simulink model "delay_brake"  (R2021a)
settings: Solver=FixedStepAuto  StartTime=0.0  StopTime=inf  FixedStep=0.05  RelTol=1e-3
undefined symbols (not defined in the file): Linear
libraries: robotlib x16
settings Model: Creator=ivory  LastModifiedBy=vanderbilt
settings SolverCC: AlgebraicLoopSolver=TrustRegion
settings OptimizationCC: EnhancedBackFolding=on  PassReuseOutputArgsAs=Individual arguments  ZeroExternalMemoryAtStartup=off  ZeroInternalMemoryAtStartup=off  MaxStackSize=64  OptimizeBlockOrder=speed  DifferentSizesBufferReuse=on  OptimizationCustomize=off  EfficientTunableParamExpr=on
settings DebuggingCC: ParameterTunabilityLossMsg=error  SFMachineParentedDataDiag=warning
settings HardwareCC: ProdBitPerPointer=32  ProdBitPerSizeT=32  ProdBitPerPtrDiffT=32  ProdLargestAtomicFloat=None  ProdIntDivRoundTo=Undefined  ProdEndianess=Unspecified  ProdWordSize=32  ProdHWDeviceType=Generic->Unspecified (assume 32-bit Generic)
settings SFSimCC: MATLABDynamicMemAlloc=off  SimTargetLang=C++
settings RTWCC: SystemTargetFile=ert.tlc  HardwareBoard=Robot Operating System (ROS)  TLCOptions="-aInlineSetEventsForThisBaseRateFcn=TLC_FALSE -aSuppressMultiTaskScheduler=TLC_FALSE  -aRateBasedStepFcn=0"  TemplateMakefile=ert_default_tmf  GenerateReport=on  Toolchain=Catkin  IncludeHyperlinkInReport=on  LaunchReport=on  TargetLang=C++  GenerateTraceInfo=on  GenerateTraceReport=on  GenerateTraceReportSl=on  GenerateTraceReportSf=on  GenerateTraceReportEml=on
settings CodeAppCC: ForceParamTrailComments=on  IgnoreCustomStorageClasses=off  OperatorAnnotations=on  SimulinkDataObjDesc=on  SFDataObjDesc=on  InsertBlockDesc=on
settings ERTTargetCC: SupportContinuousTime=on  SupportVariableSizeSignals=on

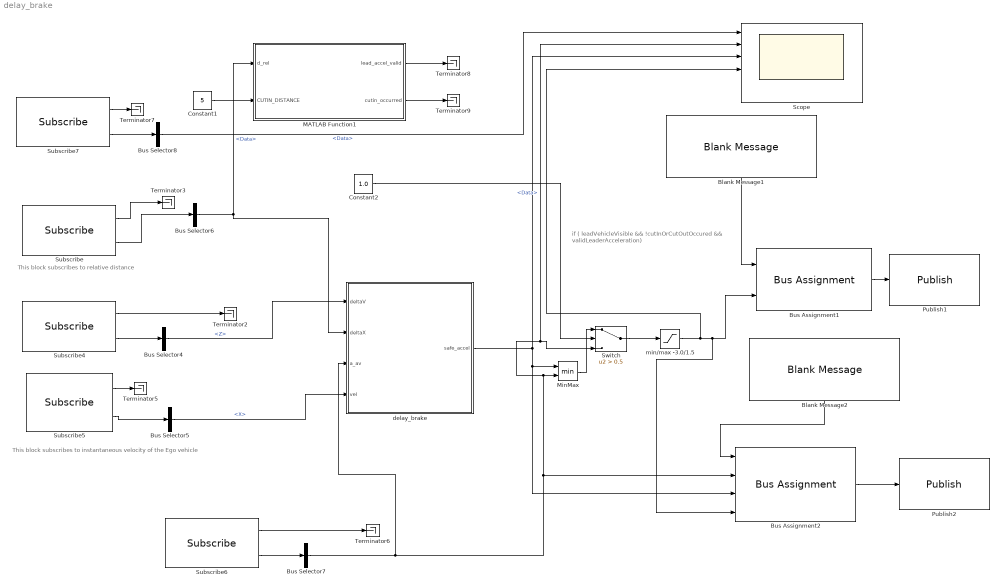
== system delay_brake ==
  note: if ( leadVehicleVisible && !cutInOrCutOutOccured && validLeaderAcceleration)
  note: This block subscribes
      | to relative distance
  note: This block subscribes to
      | instantaneous velocity of the Ego vehicle
  Blank Message1 : robotlib/Blank Message  messageClass=Message  entityType=std_msgs/Float64  messageType=std_msgs/Float64  SampleTime=inf  legacyBusStruct=off
  Blank Message2 : robotlib/Blank Message  messageClass=Message  entityType=geometry_msgs/Twist  messageType=geometry_msgs/Twist  SampleTime=inf  legacyBusStruct=off
  Bus Assignment1 : BusAssignment  AssignedSignals=Data
  Bus Assignment2 : BusAssignment  AssignedSignals=Linear.X,Linear.Y,Linear.Z
  Bus Selector4 : BusSelector  OutputSignals=Linear.Z
  Bus Selector5 : BusSelector  OutputSignals=Linear.X
  Bus Selector6 : BusSelector  OutputSignals=Data
  Bus Selector7 : BusSelector  OutputSignals=Data
  Bus Selector8 : BusSelector  OutputSignals=Data
  Constant1 : Constant  Value=5
  Constant2 : Constant  Value=1.0
  MATLAB Function1 : MATLAB Function  TreatAsAtomicUnit=on
  MinMax : MinMax  Inputs=2
  Publish1 : robotlib/Publish  topicSource=Specify your own  topic=cmd_accel  messageType=std_msgs/Float64  legacyBusStruct=off  messageQueueLength=1
  Publish2 : robotlib/Publish  topicSource=Specify your own  topic=/delay_brake/delay_brake_debug  messageType=geometry_msgs/Twist  legacyBusStruct=off  messageQueueLength=1
  Scope : Scope  NumInputPorts=6
  Subscribe : robotlib/Subscribe  topicSource=Specify your own  topic=lead_dist  messageType=std_msgs/Float64  SampleTime=-1  legacyBusStruct=off  messageQueueLength=1
  Subscribe4 : robotlib/Subscribe  topicSource=Specify your own  topic=rel_vel  messageType=geometry_msgs/Twist  SampleTime=-1  legacyBusStruct=off  messageQueueLength=1
  Subscribe5 : robotlib/Subscribe  topicSource=Specify your own  topic=vel  messageType=geometry_msgs/Twist  SampleTime=-1  legacyBusStruct=off  messageQueueLength=1
  Subscribe6 : robotlib/Subscribe  topicSource=Specify your own  topic=cmd_accel_pre  messageType=std_msgs/Float64  SampleTime=-1  legacyBusStruct=off  messageQueueLength=1
  Subscribe7 : robotlib/Subscribe  topicSource=Specify your own  topic=/car/hud/mini_car_enable  messageType=std_msgs/Bool  SampleTime=-1  legacyBusStruct=off  messageQueueLength=1
  Switch : Switch  Criteria=u2 > Threshold  Threshold=0.5
  Terminator{2..3,5..9} (7 alike) : Terminator
  delay_brake : Subsystem
  min/max -3.0/1.5 : Saturate  UpperLimit=1.5  LowerLimit=-3.0
  wires:
  Subscribe4/1 -> Terminator2/1
  Bus Selector4/1 -> delay_brake/1(deltaV)  "<Z>"
  Subscribe5/2 -> Bus Selector5/1
  Subscribe4/2 -> Bus Selector4/1
  Bus Selector5/1 -> delay_brake/4(vel)  "<X>"
  Bus Assignment1/1 -> Publish1/1
  Blank Message1/1 -> Bus Assignment1/1
  Subscribe5/1 -> Terminator5/1
  Subscribe/1 -> Terminator3/1
  Subscribe/2 -> Bus Selector6/1
  Bus Selector6/1 -> MATLAB Function1/1(d_rel), delay_brake/2(deltaX)  "<Data>"
  Subscribe6/2 -> Bus Selector7/1
  Bus Selector7/1 -> delay_brake/3(a_av), MinMax/2, Switch/3, Scope/2, Bus Assignment2/2  "<Data>"
  Subscribe6/1 -> Terminator6/1
  Subscribe7/2 -> Bus Selector8/1
  Subscribe7/1 -> Terminator7/1
  Bus Selector8/1 -> Scope/1  "<Data>"
  Constant1/1 -> MATLAB Function1/2(CUTIN_DISTANCE)
  delay_brake/1(safe_accel) -> Scope/3, Bus Assignment2/3, MinMax/1
  MinMax/1 -> Switch/1
  min/max -3.0/1.5/1 -> Scope/4, Bus Assignment2/4, Bus Assignment1/2
  Blank Message2/1 -> Bus Assignment2/1
  Bus Assignment2/1 -> Publish2/1
  MATLAB Function1/1(lead_accel_valid) -> Terminator8/1
  MATLAB Function1/2(cutin_occurred) -> Terminator9/1
  Switch/1 -> min/max -3.0/1.5/1
  Constant2/1 -> Switch/2

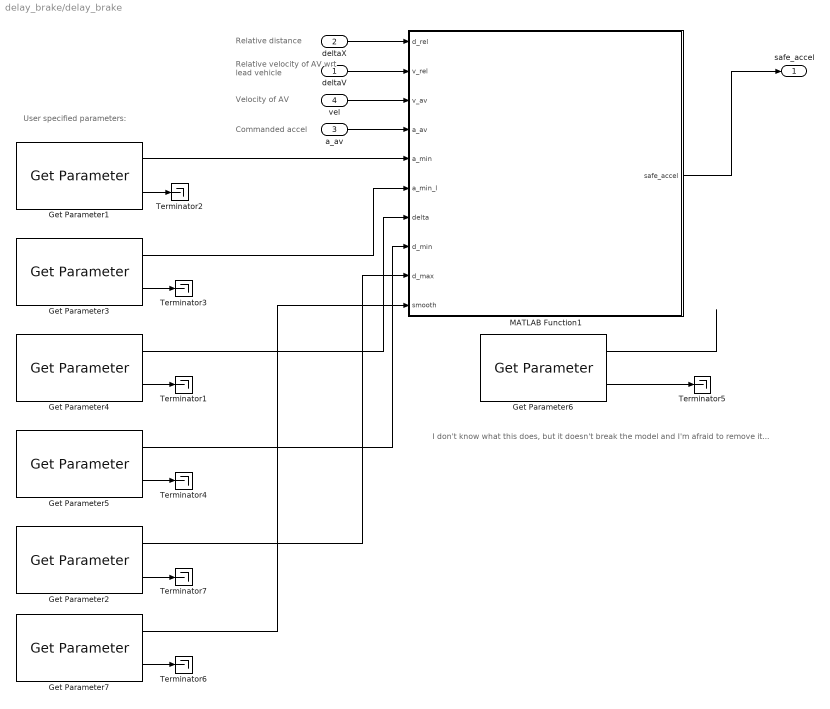
== system delay_brake/delay_brake ==
  note: I don't know what this does, but it doesn't break the model and I'm afraid to remove it...
  note: Velocity of AV
  note: Relative velocity of
      | AV wrt lead vehicle
  note: Relative distance
  note: Commanded accel
  note: User specified parameters:
  deltaV : Inport
  deltaX : Inport  Port=2
  a_av : Inport  Port=3
  vel : Inport  Port=4
  Get Parameter1 : robotlib/Get Parameter  ParameterSource=Specify your own  ParameterName=a_min  ParameterType=double  ParameterMaxArrayLength=16  ParameterInitialValue=-3.0  SampleTime=-1  ShowErrorCodeOutput=on  ModelName=delay_brake  BlockId=ParamGet_delay_brake_447
      settings: SourceProductBaseCode=RR
  Get Parameter2 : robotlib/Get Parameter  ParameterSource=Specify your own  ParameterName=d_max  ParameterType=double  ParameterMaxArrayLength=16  ParameterInitialValue=15.0  SampleTime=-1  ShowErrorCodeOutput=on  ModelName=delay_brake  BlockId=ParamGet_delay_brake_448
      settings: SourceProductBaseCode=RR
  Get Parameter3 : robotlib/Get Parameter  ParameterSource=Specify your own  ParameterName=a_min_l  ParameterType=double  ParameterMaxArrayLength=16  ParameterInitialValue=-3.0  SampleTime=-1  ShowErrorCodeOutput=on  ModelName=delay_brake  BlockId=ParamGet_delay_brake_449
      settings: SourceProductBaseCode=RR
  Get Parameter4 : robotlib/Get Parameter  ParameterSource=Specify your own  ParameterName=delta  ParameterType=double  ParameterMaxArrayLength=16  ParameterInitialValue=0.2  SampleTime=-1  ShowErrorCodeOutput=on  ModelName=delay_brake  BlockId=ParamGet_delay_brake_450
      settings: SourceProductBaseCode=RR
  Get Parameter5 : robotlib/Get Parameter  ParameterSource=Specify your own  ParameterName=d_min  ParameterType=double  ParameterMaxArrayLength=16  ParameterInitialValue=2.0  SampleTime=-1  ShowErrorCodeOutput=on  ModelName=delay_brake  BlockId=ParamGet_delay_brake_463
      settings: SourceProductBaseCode=RR
  Get Parameter6 : robotlib/Get Parameter  ParameterSource=Specify your own  ParameterName=w3  ParameterType=double  ParameterMaxArrayLength=16  ParameterInitialValue=6.0  SampleTime=-1  ShowErrorCodeOutput=on  ModelName=delay_brake  BlockId=ParamGet_delay_brake_465
      settings: SourceProductBaseCode=RR
  Get Parameter7 : robotlib/Get Parameter  ParameterSource=Specify your own  ParameterName=smooth  ParameterType=boolean  ParameterMaxArrayLength=16  ParameterInitialValue=1  SampleTime=-1  ShowErrorCodeOutput=on  ModelName=delay_brake  BlockId=ParamGet_delay_brake_529
      settings: SourceProductBaseCode=RR
  MATLAB Function1 : MATLAB Function  TreatAsAtomicUnit=on
  Terminator{1..7} (7 alike) : Terminator
  safe_accel : Outport
  wires:
  Get Parameter4/1 -> MATLAB Function1/7(delta)
  Get Parameter4/2 -> Terminator1/1
  Get Parameter2/1 -> MATLAB Function1/9(d_max)
  Get Parameter2/2 -> Terminator7/1
  Get Parameter3/2 -> Terminator3/1
  Get Parameter1/1 -> MATLAB Function1/5(a_min)
  Get Parameter1/2 -> Terminator2/1
  Get Parameter3/1 -> MATLAB Function1/6(a_min_l)
  MATLAB Function1/1(safe_accel) -> safe_accel/1
  vel/1 -> MATLAB Function1/3(v_av)
  deltaV/1 -> MATLAB Function1/2(v_rel)
  deltaX/1 -> MATLAB Function1/1(d_rel)
  Get Parameter5/2 -> Terminator4/1
  Get Parameter5/1 -> MATLAB Function1/8(d_min)
  Get Parameter6/1 -> ?
  Get Parameter6/2 -> Terminator5/1
  a_av/1 -> MATLAB Function1/4(a_av)
  Get Parameter7/2 -> Terminator6/1
  Get Parameter7/1 -> MATLAB Function1/10(smooth)

== matlab function delay_brake/MATLAB Function1 ==
  data: safe_accel output; d_rel input; v_rel input; v_av input; a_av input; a_min input; a_min_l input; delta input; d_min input; d_max input; smooth input
function safe_accel = ...
    fcn(d_rel,v_rel,v_av,a_av,a_min,a_min_l,delta,d_min,d_max,smooth)
%#codegen

% Code from Alex K.

% follower is used synonym with AV
% d_rel relative position leader follower
% v_rel relative velocity leader follower
% v_av autonomous (follower) vehicle velocity
% a_av commanded acceleration (which we might want to overwrite if not
% safe)
% a_min minimal acceleration follower (a_min<0)
% a_min_l minimal acceleration leader (a_min_l<0)
% delta reaction delay of the follower assuming that the follower drives
% for another \delta s until it can brake
% car length of the leader l
% d_min minimal saftety distance between follower and leader
% d_max safety distance for smoothing the accleration, d_max>d_min. Only
% applied if we use the smooth version of the controller
% smooth\in\{0,1\} smoothing parameter to not directly start braking as heavily as possible but braking slower between d_min and d_max
% %Derivation of the formulae:
% Computing the required distance for the follower assuming that they do not react (drive with constant speed) for delta seconds and then break as heavily as possible
% 1) computing how long it takes to stop the AV currently driving with speed v: v+amin*t=0\implies T_stop=-v/amin.
% 2) computing the space it takes to stop the vehicle then
% int_{0}^{-v/amin}v+amin*t\dd t=-v^2/amin +1/2v^2/amin=-1/2v^2/amin, thus altogether we have as distance travelled in the worst case (heavy braking)
% X=x+delta*v-1/2*v^2/amin;
% 3) same for the leader, but without delay t
%car length set to
l=3.5;
% computing leader's velocity
% vl=v_rel-v_av; % This is a typo in the original


safe_accel = a_av;

vl = v_av + v_rel;
%computing distance when both vehicles have stopped and having applied max
%decleration
X_rel =d_rel-1/2*vl.^2/a_min_l -delta*v_av+1/2*(v_av).^2/a_min -l;
if X_rel <=d_min
        %break as heavy as possible, we are almost in the region of crash given the leader starts braking crazily.
   safe_accel=a_min;
elseif smooth==1 %smoothed controller when we are close to the safety distance, we interpolate between braking maximal and not braking at all
    if X_rel >d_min && X_rel<d_max
            safe_accel= min(a_min/(d_max-d_min)*(d_max-X_rel),a_av);
    elseif X_rel>d_max
            safe_accel=a_av;
    end
elseif smooth==0 % not smoothed controller: If we are not in the dangerous area (even if we are close to it), we just use the originally commanded acceleration
            safe_accel=a_av;
end




end





% Old CBF code:

% % from the timegap filter function
% % maybe make this gain a parameter later
% % k = 0.1;
% k = k_timegap;
% %t_min = 2.0;
% t_min = timegap;
% timegap_accel = (1/t_min)*v_rel + (k/t_min)*(d_rel - t_min*v_av);
% 
% % from collision-avoid filter function
% % a potential parameter - read into the fcn now
% % s_min = 15.0;
% % a potential parameter - read into the fcn now
% % k1 = 0.5;
% % a potential parameter - read into the fcn now
% % k2 = 0.5;
% %a_max = a_l + (k1+k2)*(delta_v) + (k1*k2)*(s-s_min);
% % simplification TODO this is maybe dangerous so need to confirm
% a_l = 0;
% collision_avoid_accel = a_l + (k1+k2)*(v_rel) + (k1*k2)*(d_rel-s_min);
% 
% % now put these together
% % 	 tg_accel = time_gap_filter(v,s,delta_v)
% % 	 ca_accel = collision_avoid_filter(s,delta_v,a_l)
% % 	 return min([tg_accel,ca_accel])
% % TODO make max/min acceleration parameters.
% % safe_accel = min(1.5,max(-3.0,min(timegap_accel,collision_avoid_accel)));
% safe_accel = min(timegap_accel,collision_avoid_accel);

== matlab function delay_brake/MATLAB Function1 ==
  data: lead_accel_valid output; d_rel input; CUTIN_DISTANCE input; cutin_occurred output
function [lead_accel_valid, cutin_occurred]= fcn(d_rel,CUTIN_DISTANCE)
%#codegen

persistent relative_distance_prev;
if isempty(relative_distance_prev)
    relative_distance_prev=d_rel;
end

cutin_occurred = 1;
lead_accel_valid=1;

if( abs( relative_distance_prev - d_rel ) > CUTIN_DISTANCE )
    cutin_occurred = 1;
else
    cutin_occurred = 0;
end

relative_distance_prev = d_rel;
